simulink model "ex_22_model"  (R2014a)
settings: Solver=ode45  StartTime=0.0  StopTime=4  RelTol=1e-3
undefined symbols (not defined in the file): ki, Kp, x, y, z
settings Model: Creator=Nino  LastModifiedBy=Nino

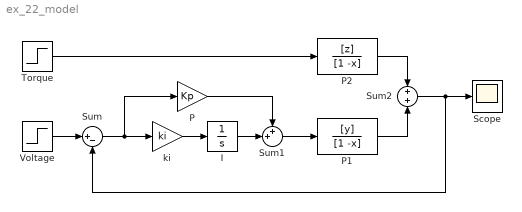
== system ex_22_model ==
  I : Integrator
  P : Gain  Gain=Kp
  P1 : TransferFcn  Numerator=[y]  Denominator=[1 -x]
  P2 : TransferFcn  Numerator=[z]  Denominator=[1 -x]
  Scope : Scope
      settings: YMin=0.9989  YMax=0.9999
  Sum : Sum  Inputs=|+-
  Sum1 : Sum  Inputs=++|
  Sum2 : Sum  Inputs=+|+
  Torque : Step  Time=2  After=0.1  SampleTime=0
  Voltage : Step  SampleTime=0
  ki : Gain  Gain=ki
  wires:
  Torque/1 -> P2/1
  P2/1 -> Sum2/1
  Sum2/1 -> Sum/2, Scope/1
  Voltage/1 -> Sum/1
  ki/1 -> I/1
  Sum/1 -> P/1, ki/1
  P/1 -> Sum1/1
  I/1 -> Sum1/2
  Sum1/1 -> P1/1
  P1/1 -> Sum2/2
